simulink model "developing_the_method"  (R2017b)
settings: Solver=VariableStepAuto  StartTime=0.0  StopTime=20  RelTol=1e-3
libraries: simulink x2
settings Model: Creator=Tom  LastModifiedBy=Tom

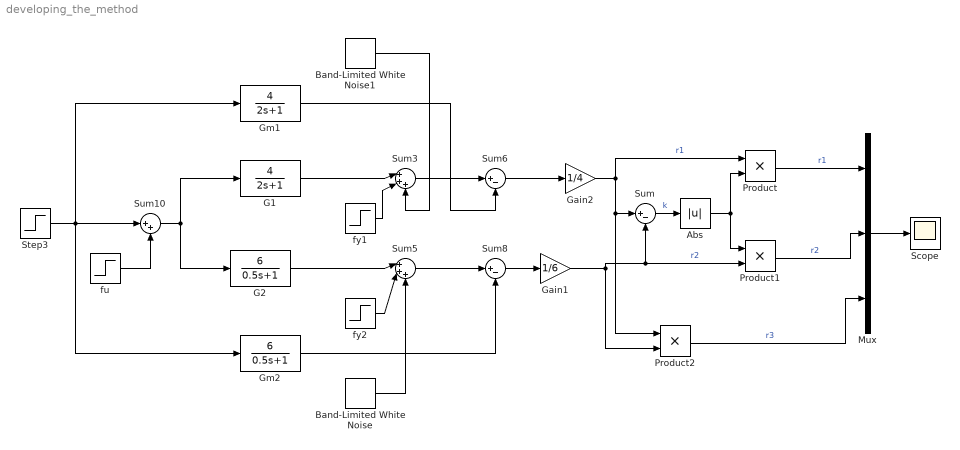
== system developing_the_method ==
  Abs : Abs
  Band-Limited White Noise : simulink/Sources/Band-Limited White Noise  Cov=[0.01]  Ts=0.025  seed=[23341]
  Band-Limited White Noise1 : simulink/Sources/Band-Limited White Noise  Cov=[0.01]  Ts=0.025  seed=[23341]
  "G1 " : TransferFcn  Numerator=[4]  Denominator=[2 1]
  G2 : TransferFcn  Numerator=[6]  Denominator=[0.5 1]
  Gain1 : Gain  Gain=1/6
  Gain2 : Gain  Gain=1/4
  Gm1 : TransferFcn  Numerator=[4]  Denominator=[2 1]
  Gm2 : TransferFcn  Numerator=[6]  Denominator=[0.5 1]
  Mux : Mux  Inputs=3
  Product : Product
  Product1 : Product
  Product2 : Product
  Scope : Scope
  Step3 : Step  Time=0  SampleTime=0
  Sum : Sum  Inputs=|+-
  Sum10 : Sum  Inputs=|++
  Sum3 : Sum  Inputs=|+++
  Sum5 : Sum  Inputs=|+++
  Sum6 : Sum  Inputs=|+-
  Sum8 : Sum  Inputs=|+-
  fu : Step  Time=5  After=0  SampleTime=0
  fy1 : Step  Time=5  After=0  SampleTime=0
  fy2 : Step  Time=5  After=0  SampleTime=0
  wires:
  fy1/1 -> Sum3/2
  fy2/1 -> Sum5/2
  G2/1 -> Sum5/1
  Step3/1 -> Gm2/1, Sum10/1, Gm1/1
  Sum10/1 -> G2/1, "G1 "/1
  fu/1 -> Sum10/2
  Sum3/1 -> Sum6/1
  Gm1/1 -> Sum6/2
  Sum6/1 -> Gain2/1
  Sum5/1 -> Sum8/1
  Sum8/1 -> Gain1/1
  Gm2/1 -> Sum8/2
  Mux/1 -> Scope/1
  Gain1/1 -> Sum/2, Product1/2, Product2/2  "r2"
  Gain2/1 -> Product/1, Product2/1, Sum/1  "r1"
  Product/1 -> Mux/1  "r1"
  Product1/1 -> Mux/2  "r2"
  Sum/1 -> Abs/1  "k"
  Abs/1 -> Product/2, Product1/1
  "G1 "/1 -> Sum3/1
  Product2/1 -> Mux/3  "r3"
  Band-Limited White Noise/1 -> Sum5/3
  Band-Limited White Noise1/1 -> Sum3/3
